simulink model "rotpentemplate_MPC"  (R2018b)
settings: Solver=ode45  StartTime=0.0  StopTime=30  RelTol=1e-3  EnableMultiTasking=on
InitFcn:
  | MPC
undefined symbols (not defined in the file or in its folder): adingain, adinoffs, daoutgain, daoutoffs, h
libraries: mpclib x1
settings Model: Creator=rbabuska  LastModifiedBy=janneke
settings DataIOCC: SaveFormat=Array  SignalLoggingName=sigsOut
settings OptimizationCC: BooleanDataType=off  ExpressionDepthLimit=2147483647  InitFltsAndDblsToZero=on  LifeSpan=inf
settings DebuggingCC: SaveWithParameterizedLinksMsg=none  SignalResolutionControl=TryResolveAllWithWarning  MultiTaskDSMMsg=warning  MultiTaskCondExecSysMsg=none  AllowSymbolicDim=off  StateNameClashWarn=warning  SFUnexpectedBacktrackingDiag=warning  SFNoUnconditionalDefaultTransitionDiag=warning  SFExecutionAtInitializationDiag=none
settings HardwareCC: ProdBitPerPointer=32  ProdBitPerSizeT=32  ProdBitPerPtrDiffT=32  ProdLargestAtomicFloat=None  ProdIntDivRoundTo=Undefined  ProdEndianess=Unspecified  ProdWordSize=32  ProdHWDeviceType=32-bit Generic  TargetUnknown=on
settings ModelReferenceCC: PropagateSignalLabelsOutOfModel=off
settings SFSimCC: SimUseLocalCustomCode=off
settings RTWCC: RTWUseLocalCustomCode=off
settings CodeAppCC: StateflowObjectComments=on
settings GRTTargetCC: TargetFcnLib=ansi_tfl_tmw.mat  TargetLangStandard=C89/C90 (ANSI)  GeneratePreprocessorConditionals=Disable all  CombineOutputUpdateFcns=off  GRTInterface=on
settings ConfigComp: CovMetricSettings=dw  CovHtmlReporting=on  CovSaveCumulativeToWorkspaceVar=on  CovSaveSingleToWorkspaceVar=on  CovExternalEMLEnable=off

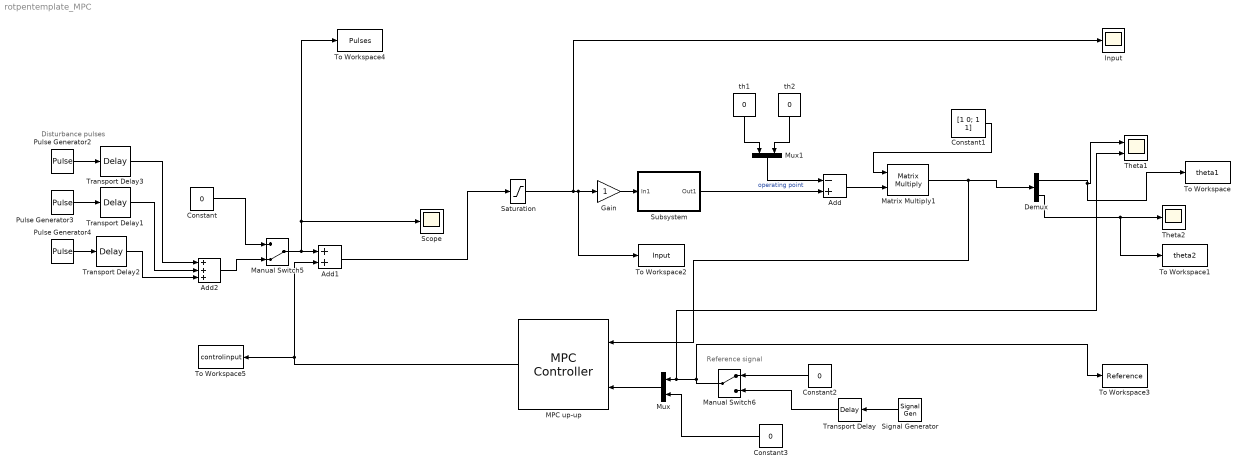
== system rotpentemplate_MPC ==
  note: Reference signal
  note: Disturbance pulses
  Add : Sum  Inputs=-+
  Add1 : Sum
  Add2 : Sum  Inputs=+++
  Constant : Constant  Value=0
  Constant1 : Constant  Value=[1 0; 1 1]
  Constant2 : Constant  Value=0
  Constant3 : Constant  Value=0
  Demux : Demux  Outputs=2
  Gain : Gain
  Input : Scope
  "MPC up-up " : mpclib/MPC Controller  SCDEnableBlockLinearizationSpecification=on  mpcobj=MPCobj_tuning  is_multiple=0  enable_value=0  return_u0=off  updateMPCinCallerWorkspace=on  md_inport=off  mv_inport=off  return_cost=off  return_mvseq=off  return_qpstatus=off  return_xseq=off  return_state=off  return_ovseq=off  state_inport=off  umin_inport=off  umax_inport=off  ymin_inport=off  ymax_inport=off  cc_inport=off  ywt_inport=off  uwt_inport=off  duwt_inport=off  rhoeps_inport=off  uref_inport=off  n_ts=0.01  n_p=10  n_mv=1  n_md=0  n_ud=0  n_mo=2  n_uo=0  BlockDataType=double  SampleTimeInherited=off  switch_inport=off
  Manual Switch5 : ManualSwitch  CurrentSetting=0
  Manual Switch6 : ManualSwitch
  Matrix Multiply1 : Product  Multiplication=Matrix(*)
  Mux : Mux  Inputs=2
  Mux1 : Mux  Inputs=2
  Pulse Generator2 : DiscretePulseGenerator  PulseType=Time based  Amplitude=0.4  Period=10
  Pulse Generator3 : DiscretePulseGenerator  PulseType=Time based  Amplitude=0.2  Period=10
  Pulse Generator4 : DiscretePulseGenerator  PulseType=Time based  Amplitude=0.2  Period=10
  Saturation : Saturate  UpperLimit=1  LowerLimit=-1
  Scope : Scope
  Signal Generator : SignalGenerator  Amplitude=0.4  Frequency=1/15
  Subsystem : Subsystem
      mask Display: disp('Rotational\nPendulum')
  Theta1 : Scope  NumInputPorts=2
  Theta2 : Scope
  To Workspace : ToWorkspace  VariableName=theta1  SaveFormat=Timeseries  SampleTime=-1
  To Workspace1 : ToWorkspace  VariableName=theta2  SaveFormat=Timeseries  SampleTime=-1
  To Workspace2 : ToWorkspace  VariableName=Input  SaveFormat=Timeseries  SampleTime=-1
  To Workspace3 : ToWorkspace  VariableName=Reference  SaveFormat=Timeseries  SampleTime=-1
  To Workspace4 : ToWorkspace  VariableName=Pulses  SaveFormat=Timeseries  SampleTime=-1
  To Workspace5 : ToWorkspace  VariableName=controlinput  SaveFormat=Timeseries  SampleTime=-1
  Transport Delay : TransportDelay  DelayTime=5
  Transport Delay1 : TransportDelay  DelayTime=17
  Transport Delay2 : TransportDelay  DelayTime=27
  Transport Delay3 : TransportDelay  DelayTime=7
  th1 : Constant  Value=0
  th2 : Constant  Value=0
  wires:
  Saturation/1 -> Gain/1, To Workspace2/1, Input/1
  Subsystem/1(Out1) -> Add/2
  Demux/1 -> To Workspace/1, Theta1/1
  Demux/2 -> To Workspace1/1, Theta2/1
  Add/1 -> Matrix Multiply1/2
  Constant1/1 -> Matrix Multiply1/1
  Constant3/1 -> Mux/2
  Mux/1 -> "MPC up-up "/2
  Matrix Multiply1/1 -> "MPC up-up "/1, Demux/1
  Gain/1 -> Subsystem/1(In1)
  Mux1/1 -> Add/1  "operating point"
  th2/1 -> Mux1/2
  th1/1 -> Mux1/1
  "MPC up-up "/1 -> To Workspace5/1, Add1/2
  Signal Generator/1 -> Transport Delay/1
  Manual Switch6/1 -> To Workspace3/1, Theta1/2, Mux/1
  Add1/1 -> Saturation/1
  Pulse Generator2/1 -> Transport Delay3/1
  Pulse Generator3/1 -> Transport Delay1/1
  Transport Delay1/1 -> Add2/2
  Pulse Generator4/1 -> Transport Delay2/1
  Transport Delay2/1 -> Add2/3
  Transport Delay3/1 -> Add2/1
  Manual Switch5/1 -> To Workspace4/1, Scope/1, Add1/1
  Add2/1 -> Manual Switch5/2
  Constant/1 -> Manual Switch5/1
  Transport Delay/1 -> Manual Switch6/2
  Constant2/1 -> Manual Switch6/1

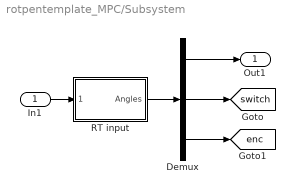
== system rotpentemplate_MPC/Subsystem ==
  In1 : Inport
  Demux : Demux  Outputs=[2 4 1]
  RT input : Subsystem  mask{Ts=h, channels=[6 7]}
      mask prompts: Ts "Sample time [s]:"; channels "Channels to read (e.g., [6 7])"
      mask init:
      | hwinit;
      | 
      | % initialize FPGA
      | fugihandle = fugiboard('Open', 'Pendulum1');
      | fugihandle.WatchdogTimeout = 0.5;
      | fugiboard('SetParams', fugihandle);
      | fugiboard('Write', fugihandle, 0, 0, 0, 0);  % dummy write to sync interface board
      | fugiboard('Write', fugihandle, 5, 1, 0, 0);  % reset position, activate relay
      | data = fugiboard('Read', fugihandle);        % get version info from FPGA
      | % model = bitshift(data(1), -5); 
      | % version = bitand(data(1), 31);
      | % disp(sprintf('FPGA setup %d, version %d', model, version)); % for the B&P it should say 1 1, or else there is a problem
      | fugiboard('Write', fugihandle, 0, 1, 0, 0);  % end reset
      | pause(0.1);                         % give relay some time to respond
      mask Display: disp('Rotational\nPendulum')
  Out1 : Outport
  tag scope: enc=global, switch=global
  wires:
  RT input/1(Angles) -> Demux/1
  Demux/1 -> Out1/1
  Demux/2 -> [switch]
  Demux/3 -> [enc]
  In1/1 -> RT input/1(Motors)

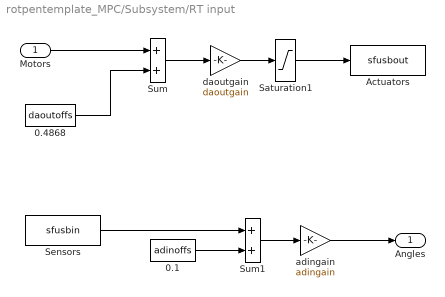
== system rotpentemplate_MPC/Subsystem/RT input ==
  Motors : Inport
  0.1 : Constant  Value=adinoffs
  0.4868 : Constant  Value=daoutoffs
  Actuators : S-Function  FunctionName=sfusbout  Parameters=Ts, fugihandle  SFunctionDeploymentMode=off  EnableBusSupport=off
  Saturation1 : Saturate  UpperLimit=10  LowerLimit=-10
  Sensors : S-Function  FunctionName=sfusbin  Parameters=Ts, fugihandle, channels  SFunctionDeploymentMode=off  EnableBusSupport=off
  Sum : Sum  SaturateOnIntegerOverflow=on  InputSameDT=on  OutDataTypeStr=Inherit: Same as first input
  Sum1 : Sum  SaturateOnIntegerOverflow=on  InputSameDT=on  OutDataTypeStr=Inherit: Same as first input
  adingain : Gain  Gain=adingain  SaturateOnIntegerOverflow=on  OutDataTypeStr=Inherit: Same as input  ParamDataTypeStr=Inherit: Same as input
  daoutgain : Gain  Gain=daoutgain  SaturateOnIntegerOverflow=on  OutDataTypeStr=Inherit: Same as input  ParamDataTypeStr=Inherit: Same as input
  Angles : Outport
  wires:
  Sum/1 -> daoutgain/1
  0.4868/1 -> Sum/2
  Motors/1 -> Sum/1
  Sum1/1 -> adingain/1
  0.1/1 -> Sum1/2
  adingain/1 -> Angles/1
  Saturation1/1 -> Actuators/1
  daoutgain/1 -> Saturation1/1
  Sensors/1 -> Sum1/1
